simulink model "Laba2post"  (R2017b)
settings: Solver=VariableStepAuto  StartTime=0.0  StopTime=100000  RelTol=1e-3
values from neighbouring files (symbols this model uses):
  Fg1 = m1*g*sin(alpha)    [lab2_data.m]
  Fg2 = m2*g*sin(alpha)    [lab2_data.m]
  kdmp = 1.5    [Labdata.m]    (also in lab2_data.m = 2)
  ksp = 12    [Labdata.m]    (also in lab2_data.m = 20)
  m1 = 200    [lab2_data.m]
  m2 = 50    [lab2_data.m]
  wr = sqrt(ksp*M/m1/m2)    [lab2_data.m]
libraries: fl_lib x10, nesl_utility x9
settings Model: Creator=Aleksandr  LastModifiedBy=Aleksandr

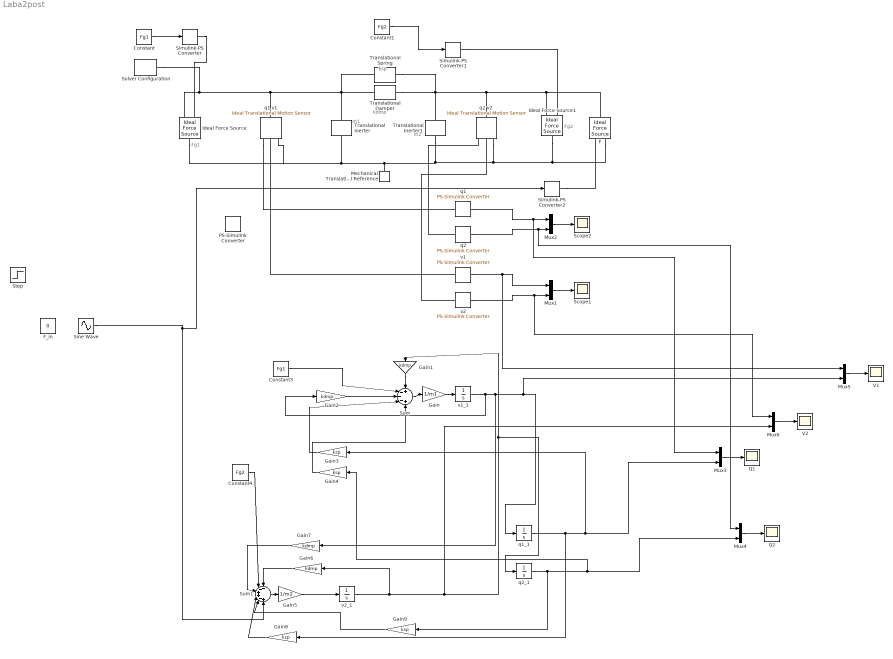
== system Laba2post ==
  note: Fg2
  note: m2
  note: m1
  note: kdmp
  note: Fg1
  note: ksp
  Constant : Constant  Value=Fg1
  Constant1 : Constant  Value=Fg2
  Constant3 : Constant  Value=Fg1
  Constant4 : Constant  Value=Fg2
  F : fl_lib/Mechanical/Mechanical Sources/Ideal Force Source
  F_in : Constant  Value=0
  Gain : Gain  Gain=1/m1
  Gain{1..2,6..7} (4 alike) : Gain  Gain=kdmp
  Gain{3..4,8..9} (4 alike) : Gain  Gain=ksp
  Gain5 : Gain  Gain=1/m2
  Ideal Force Source : fl_lib/Mechanical/Mechanical Sources/Ideal Force Source
  Ideal Force Source1 : fl_lib/Mechanical/Mechanical Sources/Ideal Force Source
  Mechanical Translational Reference : fl_lib/Mechanical/Translational Elements/Mechanical Translational Reference
  Mux{1..6} (6 alike) : Mux  Inputs=2
  PS-Simulink Converter : nesl_utility/PS-Simulink Converter  PhysicalDomain=network_engine_domain  SubClassName=ps_output  LeftPortType=input  RightPortType=output  PseudoPeriodic=off  Frequencies=[]  Unit=1  AffineConversion=off
  Q1 : Scope
  Q2 : Scope
  Scope1 : Scope
  Scope2 : Scope
  Simulink-PS Converter : nesl_utility/Simulink-PS Converter  PhysicalDomain=network_engine_domain  SubClassName=ps_input  LeftPortType=input  RightPortType=output  PseudoPeriodic=off  Frequencies=[]  NoiseDistribution=none  NoiseParameters=[]  Unit=1  AffineConversion=off  FilteringAndDerivatives=provide  SimscapeFilterOrder=1  InputFilterTimeConstant=0.001  UdotUserProvided=0
  Simulink-PS Converter1 : nesl_utility/Simulink-PS Converter  PhysicalDomain=network_engine_domain  SubClassName=ps_input  LeftPortType=input  RightPortType=output  PseudoPeriodic=off  Frequencies=[]  NoiseDistribution=none  NoiseParameters=[]  Unit=1  AffineConversion=off  FilteringAndDerivatives=provide  SimscapeFilterOrder=1  InputFilterTimeConstant=0.001  UdotUserProvided=0
  Simulink-PS Converter2 : nesl_utility/Simulink-PS Converter  PhysicalDomain=network_engine_domain  SubClassName=ps_input  LeftPortType=input  RightPortType=output  PseudoPeriodic=off  Frequencies=[]  NoiseDistribution=none  NoiseParameters=[]  Unit=1  AffineConversion=off  FilteringAndDerivatives=provide  SimscapeFilterOrder=1  InputFilterTimeConstant=0.001  UdotUserProvided=0
  Sine Wave : Sin  Amplitude=100  Bias=1  Frequency=wr*1.5  SampleTime=0
  Solver Configuration : nesl_utility/Solver Configuration  PhysicalDomain=network_engine_domain  SubClassName=solver  LeftPortType=input  RightPortType=generic  Accelerate=off  Tones=[]  Harmonics=[]  SimulateNoise=off  Profile=off  UseLocalSampling=off  EnableSwitchedLinearOptims=on  FrequencyDomain=off  UseCCode=off  RelTol=0.001  AbsTol=1e-06  MinStep=1e-09  ToWorkspace=off  RevertToSquareIcSolve=off  NumHomotopyIterations=100  PhasorMode=off  PhasorModeNumHarmonics=1  DoDC=off  ResidualTolerance=1e-09  UseLocalSolver=off  LocalSolverChoice=NE_BACKWARD_EULER_ADVANCER  LocalSolverSampleTime=0.001  DoFixedCost=off  MaxNonlinIter=3  MaxModeIter=2  LinearAlgebra=Sparse  DelaysMemoryBudget=1024  AutomaticFiltering=on  FilteringTimeConstant=0.001
  Step : Step  Before=(Fg1+Fg2)*5  After=0  SampleTime=0
  Sum : Sum  Inputs=+---+
  Sum1 : Sum  Inputs=--++-+
  Translational Inerter : fl_lib/Mechanical/Translational Elements/Translational Inerter  B=m1 kg  v_specify=off  v_priority=High  v=3 m/s  v_nominal_specify=off  v_nominal_unit=m/s  v_nominal_value=1  f_specify=off  f_priority=None  f=0 N  f_nominal_specify=off  f_nominal_unit=N  f_nominal_value=1
      settings: SourceProductName=Simscape  SourceProductBaseCode=SS
  Translational Inerter1 : fl_lib/Mechanical/Translational Elements/Translational Inerter  B=m2 kg  v_specify=off  v_priority=High  v=0 m/s  v_nominal_specify=off  v_nominal_unit=m/s  v_nominal_value=1  f_specify=off  f_priority=None  f=0 N  f_nominal_specify=off  f_nominal_unit=N  f_nominal_value=1
      settings: SourceProductName=Simscape  SourceProductBaseCode=SS
  Translational Damper : fl_lib/Mechanical/Translational Elements/Translational Damper  D=kdmp N/(m/s)  v_specify=off  v_priority=None  v=0 m/s  v_nominal_specify=off  v_nominal_unit=m/s  v_nominal_value=1  f_specify=off  f_priority=None  f=0 N  f_nominal_specify=off  f_nominal_unit=N  f_nominal_value=1
  Translational Spring : fl_lib/Mechanical/Translational Elements/Translational Spring  spr_rate=ksp N/m  v_specify=off  v_priority=None  v=0 m/s  v_nominal_specify=off  v_nominal_unit=m/s  v_nominal_value=1  f_specify=off  f_priority=None  f=0 N  f_nominal_specify=off  f_nominal_unit=N  f_nominal_value=1  x_specify=off  x_priority=High  x=0.1 m  x_nominal_specify=off  x_nominal_unit=m  x_nominal_value=1
  V1 : Scope
  V2 : Scope
  q1 : nesl_utility/PS-Simulink Converter  PhysicalDomain=network_engine_domain  SubClassName=ps_output  LeftPortType=input  RightPortType=output  PseudoPeriodic=off  Frequencies=[]  Unit=1  AffineConversion=off
  q1 v1 : fl_lib/Mechanical/Mechanical Sensors/Ideal Translational Motion Sensor  offset=0 m
  q1_1 : Integrator
  q2 : nesl_utility/PS-Simulink Converter  PhysicalDomain=network_engine_domain  SubClassName=ps_output  LeftPortType=input  RightPortType=output  PseudoPeriodic=off  Frequencies=[]  Unit=1  AffineConversion=off
  q2 v2 : fl_lib/Mechanical/Mechanical Sensors/Ideal Translational Motion Sensor  offset=0 m
  q2_1 : Integrator
  v1 : nesl_utility/PS-Simulink Converter  PhysicalDomain=network_engine_domain  SubClassName=ps_output  LeftPortType=input  RightPortType=output  PseudoPeriodic=off  Frequencies=[]  Unit=1  AffineConversion=off
  v1_1 : Integrator
  v2 : nesl_utility/PS-Simulink Converter  PhysicalDomain=network_engine_domain  SubClassName=ps_output  LeftPortType=input  RightPortType=output  PseudoPeriodic=off  Frequencies=[]  Unit=1  AffineConversion=off
  v2_1 : Integrator
  wires:
  Constant1/1 -> Simulink-PS Converter1/1
  Constant/1 -> Simulink-PS Converter/1
  Sine Wave/1 -> Sum1/6, Simulink-PS Converter2/1
  Mux1/1 -> Scope1/1
  v1/1 -> Mux5/1, Mux1/1
  v2/1 -> Mux6/1, Mux1/2
  q2/1 -> Mux4/1, Mux2/2
  Mux2/1 -> Scope2/1
  q1/1 -> Mux3/1, Mux2/1
  v2_1/1 -> Gain6/1, Mux6/2, Gain1/1, q2_1/1
  v1_1/1 -> Gain2/1, Gain7/1, Mux5/2, q1_1/1
  Mux3/1 -> Q1/1
  q1_1/1 -> Gain8/1, Gain3/1, Mux3/2
  Mux4/1 -> Q2/1
  q2_1/1 -> Gain9/1, Gain4/1, Mux4/2
  Gain/1 -> v1_1/1
  Sum/1 -> Gain/1
  Gain1/1 -> Sum/1
  Constant3/1 -> Sum/2
  Gain2/1 -> Sum/3
  Gain3/1 -> Sum/4
  Gain4/1 -> Sum/5
  Sum1/1 -> Gain5/1
  Gain5/1 -> v2_1/1
  Gain6/1 -> Sum1/1
  Constant4/1 -> Sum1/2
  Gain7/1 -> Sum1/3
  Gain8/1 -> Sum1/4
  Gain9/1 -> Sum1/5
  Mux6/1 -> V2/1
  Mux5/1 -> V1/1
  connections:
  Ideal Force Source1/RConn2 -- F/LConn1 -- Translational Spring/RConn1 -- Translational Inerter1/LConn1 -- Translational Damper/RConn1 -- q2 v2/LConn1
  Ideal Force Source/RConn2 -- Translational Inerter/LConn1 -- Translational Damper/LConn1 -- Translational Spring/LConn1 -- q1 v1/LConn1 -- Solver Configuration/RConn1
  Ideal Force Source1/LConn1 -- F/RConn2 -- Mechanical Translational Reference/LConn1 -- q1 v1/RConn1 -- Ideal Force Source/LConn1 -- Translational Inerter/RConn1 -- Translational Inerter1/RConn1 -- q2 v2/RConn1
  Simulink-PS Converter1/RConn1 -- Ideal Force Source1/RConn1
  Simulink-PS Converter/RConn1 -- Ideal Force Source/RConn1
  Simulink-PS Converter2/RConn1 -- F/RConn1
  q1 v1/RConn3 -- q1/LConn1
  q2/LConn1 -- q2 v2/RConn3
  v1/LConn1 -- q1 v1/RConn2
  v2/LConn1 -- q2 v2/RConn2
